simulink model "MPPT_Buck"  (R2022a)
settings: Solver=VariableStepAuto  StartTime=0.0  StopTime=1  RelTol=1e-3
values from neighbouring files (symbols this model uses):
  L = 100e-6    (= 0.0001)    [Boost_Setup.m]
undefined symbols (not defined in the file or in its folder): solarPlant
libraries: spsSeriesRLCBranchLib x4, spsCurrentMeasurementLib x2, slpidlib x2, spsFirstOrderFilterLib x2, spsMosfetLib x2, spsSawtoothGeneratorLib x2, simulink x2, spsMultimeterLib x1, spsPVArrayLib x1, spsVoltageMeasurementLib x1, spspowerguiLib x1
settings Model: Creator=pclem  LastModifiedBy=fion
settings SolverCC: AlgebraicLoopSolver=TrustRegion
settings DebuggingCC: SFMachineParentedDataDiag=warning
settings RTWCC: DLArmComputeVersion=19.05

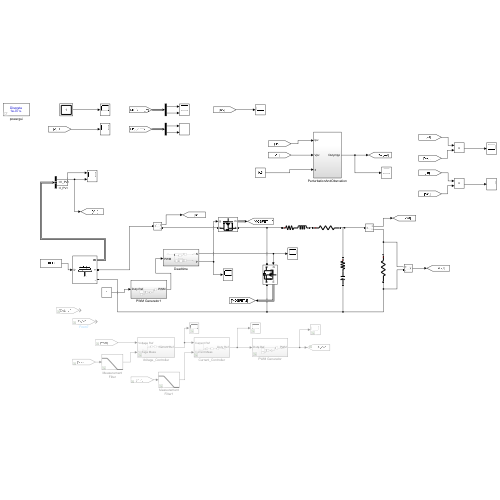
[thumbnail: Simulink's stored preview of the top-level diagram]
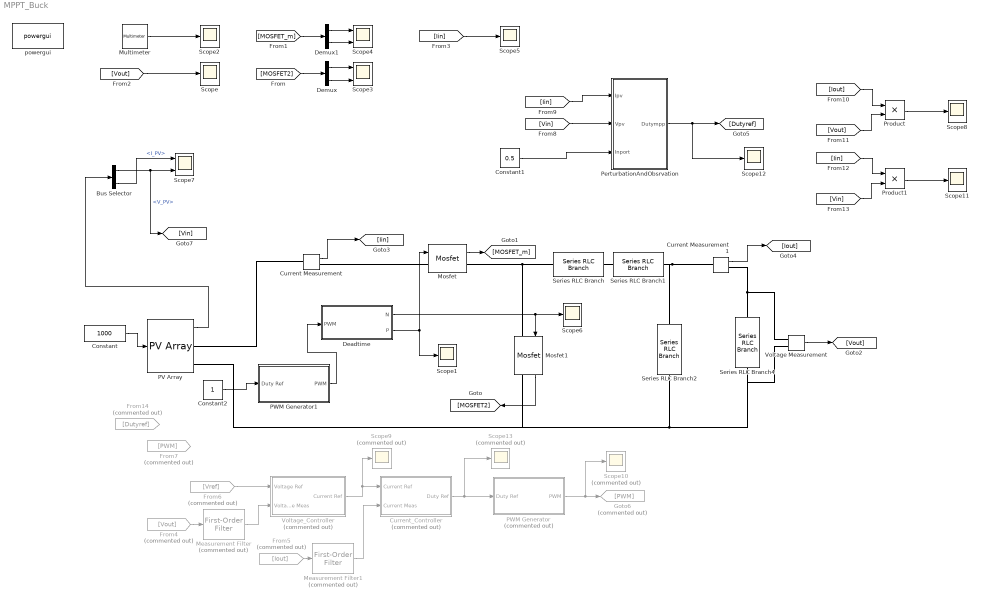
== system MPPT_Buck ==
  Bus Selector : BusSelector  OutputSignals=V_PV,I_PV
  Constant : Constant  Value=1000
  Constant1 : Constant  Value=0.5
  Constant2 : Constant
  Current Measurement : spsCurrentMeasurementLib/Current Measurement  PhasorSimulation=off  OutputType=Complex  PSBequivalent=0
  Current Measurement1 : spsCurrentMeasurementLib/Current Measurement  PhasorSimulation=off  OutputType=Complex  PSBequivalent=0
  Current_Controller : Subsystem  Commented=on
  Deadtime : Subsystem
  Demux : Demux  Outputs=2
  Demux1 : Demux  Outputs=2
  From14 : From  Commented=on  GotoTag=Dutyref
  From4 : From  Commented=on  GotoTag=Vout
  From5 : From  Commented=on  GotoTag=Iout
  From6 : From  Commented=on  GotoTag=Vref
  From7 : From  Commented=on  GotoTag=PWM
  Goto6 : Goto  Commented=on  GotoTag=PWM
  Measurement Filter : spsFirstOrderFilterLib/First-Order Filter  Commented=on  FilterType=Lowpass  Tc=10000*2.2e-9  Ts=0  Initialize=on  Vac_Init=[0, 0, 0]  Vdc_Init=0  PlotResponse=off  FreqRange="[0,  100e3,  100]"
  Measurement Filter1 : spsFirstOrderFilterLib/First-Order Filter  Commented=on  FilterType=Lowpass  Tc=10000*2.2e-9  Ts=0  Initialize=on  Vac_Init=[0, 0, 0]  Vdc_Init=0  PlotResponse=off  FreqRange="[0,  100e3,  100]"
  Mosfet : spsMosfetLib/Mosfet  Ron=0.136  Lon=0  Rd=0.01  Vfd=1.1  IC=0  Rs=1e9  Cs=inf  Measurements=on
  Mosfet1 : spsMosfetLib/Mosfet  Ron=0.136  Lon=0  Rd=0.01  Vfd=1.1  IC=0  Rs=1e9  Cs=inf  Measurements=on
  Multimeter : spsMultimeterLib/Multimeter  L=5  sel=3  yselected={}  Gain=1  OutputType=Complex  PlotAtSimulationStop=off  PhasorSimulation=off
  PV Array : spsPVArrayLib/PV Array  Npar=2  Nser=2  PlotType=array @ 1000 W/m2 & specified temperatures  S_vec="[ 1000  500  100 ]"  Temp_C_vec="[ 45 25  ]"  ModuleName=User-defined  PlotWhenSelected=off  Pm=1.0215  Ncell=2  Voc=5.7  Isc=0.24  Vm=4.5  Im=0.227  beta_Voc_pc=-0.45  alpha_Isc_pc=0.1  beta_Voc=-0.02565  alpha_Isc=0.00024  IL=0.24235  I0=1.5749e-15  nI=3  Rsh=692.3081  Rs=0.0049096  RobustModel=on  RobustCellTemperature=25  BAL=on  Tc=1e-6  Tfilter=5e-5
  PWM Generator : Subsystem  Commented=on
  PWM Generator1 : Subsystem
  PerturbationAndObsrvation : Subsystem  VariantControl=perturbationAndObservation
  Product : Product
  Product1 : Product
  Scope{,1..2,5..6,8,11..12} (8 alike) : Scope
  Scope10 : Scope  Commented=on
  Scope13 : Scope  Commented=on
  Scope3 : Scope  NumInputPorts=2
  Scope4 : Scope  NumInputPorts=2
  Scope7 : Scope  NumInputPorts=2
  Scope9 : Scope  Commented=on
  Series RLC Branch : spsSeriesRLCBranchLib/Series RLC Branch  LConnTagsString=__new0  RConnTagsString=__new0  BranchType=RL  Resistance=25e-3  Inductance=100e-6  SetiL0=off  InitialCurrent=0  Capacitance=1e-6  Setx0=off  InitialVoltage=0  Measurements=Branch current
  Series RLC Branch1 : spsSeriesRLCBranchLib/Series RLC Branch  LConnTagsString=__new0  RConnTagsString=__new0  BranchType=R  Resistance=0.1  Inductance=L  SetiL0=off  InitialCurrent=0  Capacitance=1e-6  Setx0=off  InitialVoltage=0  Measurements=Branch current
  Series RLC Branch2 : spsSeriesRLCBranchLib/Series RLC Branch  LConnTagsString=__new0  RConnTagsString=__new0  BranchType=RC  Resistance=0.1114  Inductance=1e-3  SetiL0=off  InitialCurrent=0  Capacitance=1000e-6  Setx0=off  InitialVoltage=0  Measurements=Branch voltage
  Series RLC Branch4 : spsSeriesRLCBranchLib/Series RLC Branch  LConnTagsString=__new0  RConnTagsString=__new0  BranchType=R  Resistance=10  Inductance=1e-3  SetiL0=off  InitialCurrent=0  Capacitance=1e-6  Setx0=off  InitialVoltage=0  Measurements=Branch voltage and current
  Voltage Measurement : spsVoltageMeasurementLib/Voltage Measurement  PhasorSimulation=off  OutputType=Complex  PSBequivalent=0
  Voltage_Controller : Subsystem  Commented=on
  powergui : spspowerguiLib/powergui  Priority=1  SimulationMode=Discrete  SampleTime=1e-7  frequency=60  Iterations=50  frequencyindice=0  Pbase=100e6  ErrMax=1e-4  UnitsV=kV  UnitsW=MW  buscounter=0  FunctionMessages=off  echomessages=off  EnableUseOfTLC=off  CurrentSourceSwitches=off  DisableSnubberDevices=off  DisableRonSwitches=off  DisableVfSwitches=off  DisplayEquations=off  AutomaticDiscreteSolvers=off  SolverType=Tustin/Backward Euler (TBE)  Interpol=off  ExternalGateDelay=off  methode=off  Ts=100  x0status=blocks  SPID=on  SwTol=0  HookPort=off  NonlinearTolerance=1e-4  nMaxIteration=100  ContinueOnMaxIteration=off  RestoreLinks=warning  ResistiveCurrentMeasurement=off  Frange=[0:2:500]  Ylog=off  Xlog=on  ShowGrid=off  save=off  variable=ZData  structure=0  ZoomFFT=off  StartTime=0.0  cycles=1  DisplayStyle=1  fundamental=60  FreqAxis=off  MaxFrequency=1000  frequencyindicesteady=1  RmsSteady=1  display=off
  wires:
  Multimeter/1 -> Scope2/1
  [Vout] -> Scope/1
  Mosfet/1 -> [MOSFET_m]
  Demux/2 -> Scope3/2
  Demux/1 -> Scope3/1
  [MOSFET2] -> Demux/1
  [MOSFET_m] -> Demux1/1
  Demux1/1 -> Scope4/1
  Demux1/2 -> Scope4/2
  Voltage Measurement/1 -> [Vout]
  Mosfet1/1 -> [MOSFET2]
  Current Measurement/1 -> [Iin]
  [Iin] -> Scope5/1
  Deadtime/2(P) -> Scope1/1, Mosfet/1
  Deadtime/1(N) -> Mosfet1/1, Scope6/1
  Bus Selector/2 -> Scope7/1  "<I_PV>"
  PV Array/1 -> Bus Selector/1
  Bus Selector/1 -> [Vin], Scope7/2  "<V_PV>"
  Constant/1 -> PV Array/1
  Current Measurement1/1 -> [Iout]
  Current_Controller/1(Duty Ref) -> Scope13/1, PWM Generator/1(Duty Ref)
  From5/1 -> Measurement Filter1/1
  Measurement Filter/1 -> Voltage_Controller/2(Voltage Meas)
  Voltage_Controller/1(Current Ref) -> Scope9/1, Current_Controller/1(Current Ref)
  Measurement Filter1/1 -> Current_Controller/2(Current Meas)
  PWM Generator/1(PWM) -> Scope10/1, Goto6/1
  From4/1 -> Measurement Filter/1
  From6/1 -> Voltage_Controller/1(Voltage Ref)
  [Vin] -> PerturbationAndObsrvation/2(Vpv)
  [Iout] -> Product/1
  [Vout] -> Product/2
  Product/1 -> Scope8/1
  Product1/1 -> Scope11/1
  [Vin] -> Product1/2
  [Iin] -> Product1/1
  [Iin] -> PerturbationAndObsrvation/1(Ipv)
  PerturbationAndObsrvation/1(Dutympp) -> Scope12/1, [Dutyref]
  PWM Generator1/1(PWM) -> Deadtime/1(PWM)
  Constant1/1 -> PerturbationAndObsrvation/3(Inport)
  Constant2/1 -> PWM Generator1/1(Duty Ref)
  connections:
  Voltage Measurement/LConn2 -- Series RLC Branch4/RConn1 -- PV Array/RConn2 -- Mosfet1/RConn1 -- Series RLC Branch2/RConn1
  Series RLC Branch1/LConn1 -- Series RLC Branch/RConn1
  Series RLC Branch/LConn1 -- Mosfet/RConn1 -- Mosfet1/LConn1
  Current Measurement/RConn1 -- Mosfet/LConn1
  Current Measurement1/LConn1 -- Series RLC Branch1/RConn1 -- Series RLC Branch2/LConn1
  Voltage Measurement/LConn1 -- Current Measurement1/RConn1 -- Series RLC Branch4/LConn1
  PV Array/RConn1 -- Current Measurement/LConn1

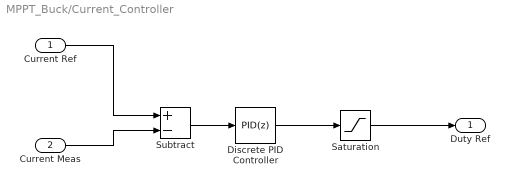
== system MPPT_Buck/Current_Controller ==
  Current Ref : Inport
  Current Meas : Inport  Port=2
  Discrete PID Controller : slpidlib/PID Controller  Controller=PID  Form=Parallel  TimeDomain=Discrete-time  UseExternalTs=off  SampleTime=1/1000  IntegratorMethod=Forward Euler  FilterMethod=Forward Euler  ControllerParametersSource=internal  P=0.02512  I=39.4  UseKiTs=off  D=0  N=100  UseFilter=off  TunerSelectOption=Transfer Function Based (PID Tuner App)  InitialConditionSource=internal  InitialConditionForIntegrator=0  InitialConditionForFilter=0  DifferentiatorICPrevScaledInput=0  ExternalReset=none  TrackingMode=off  Kt=1  LimitOutput=off  SatLimitsSource=internal  UpperSaturationLimit=inf  LowerSaturationLimit=-inf  LinearizeAsGain=off  AntiWindupMode=none  Kb=1  POutMin=[]  POutMax=[]  IOutMin=[]  IOutMax=[]  DOutMin=[]  DOutMax=[]  NOutMin=[]  NOutMax=[]  SumOutMin=[]  SumOutMax=[]  SaturationOutMin=[]  SaturationOutMax=[]  PParamMin=[]  PParamMax=[]  IParamMin=[]  IParamMax=[]  DParamMin=[]  DParamMax=[]  NParamMin=[]  NParamMax=[]  KbParamMin=[]  KbParamMax=[]  KtParamMin=[]  KtParamMax=[]  KbOutMin=[]  KbOutMax=[]  KtOutMin=[]  KtOutMax=[]  IntegratorOutMin=[]  IntegratorOutMax=[]  FilterOutMin=[]  FilterOutMax=[]  SumI1OutMin=[]  SumI1OutMax=[]  SumI2OutMin=[]  SumI2OutMax=[]  SumI3OutMin=[]  SumI3OutMax=[]  SumI4OutMin=[]  SumI4OutMax=[]  SumDOutMin=[]  SumDOutMax=[]  DifferentiatorOutMin=[]  DifferentiatorOutMax=[]  FilterDiffOutCoefMin=[]  FilterDiffOutCoefMax=[]  ReciprocalOutMin=[]  ReciprocalOutMax=[]  SumDenOutMin=[]  SumDenOutMax=[]  SumNumOutMin=[]  SumNumOutMax=[]  DivideOutMin=[]  DivideOutMax=[]  UdiffTsProdOutMin=[]  UdiffTsProdOutMax=[]  NTsProdOutMin=[]  NTsProdOutMax=[]  UintegralTsProdOutMin=[]  UintegralTsProdOutMax=[]  UngainTsProdOutMin=[]  UngainTsProdOutMax=[]  IntegratorContinuousStateAttributes=''  IntegratorStateMustResolveToSignalObject=off  IntegratorRTWStateStorageClass=Auto  FilterContinuousStateAttributes=''  FilterStateMustResolveToSignalObject=off  FilterRTWStateStorageClass=Auto  ParallelPVariant=InternalParameters  IdealPVariant=Disabled  IVariant=InternalParameters  DVariant=InternalParameters  IntegratorVariant=Discrete  SatVariant=Disabled  AWVariant=Passthrough  PCopyVariant=Disabled  TRVariant=Disabled  FdbkBlocksVariant=Forward  IdealPFdbkVariant=Disabled  SatFdbkVariant=Disabled  DerivativeFilterVariant=Differentiator  NVariant=Passthrough  NCopyVariant=Disabled_SignalSpec  FilterICVariant=InternalICsDifferentiator  IntegratorICVariant=InternalICs  ExternalResetVariant=Disabled  TRSumVariant=Passthrough  SumFdbkVariant=Disabled  SumVariant=Sum_PID  TsampFilterVariant=InternalTs  TsampNgainVariant=Passthrough  TsampIntegralVariant=Passthrough  ExternalSaturationOutDataTypeStr=Inherit: Same as second input  aMode=0
  Saturation : Saturate  UpperLimit=0.98  LowerLimit=0.02
  Subtract : Sum  Inputs=+-
  Duty Ref : Outport
  wires:
  Subtract/1 -> Discrete PID Controller/1
  Saturation/1 -> Duty Ref/1
  Current Meas/1 -> Subtract/2
  Discrete PID Controller/1 -> Saturation/1
  Current Ref/1 -> Subtract/1

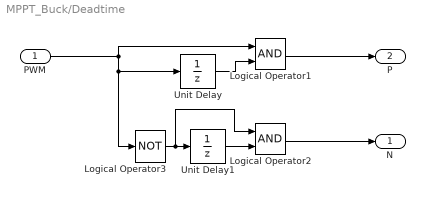
== system MPPT_Buck/Deadtime ==
  PWM : Inport
  Logical Operator1 : Logic  AllPortsSameDT=off  OutDataTypeStr=boolean
  Logical Operator2 : Logic  AllPortsSameDT=off  OutDataTypeStr=boolean
  Logical Operator3 : Logic  Operator=NOT  AllPortsSameDT=off  OutDataTypeStr=boolean
  Unit Delay : UnitDelay  SampleTime=-1  HasFrameUpgradeWarning=on
  Unit Delay1 : UnitDelay  SampleTime=-1  HasFrameUpgradeWarning=on
  N : Outport
  P : Outport  Port=2
  wires:
  Logical Operator1/1 -> P/1
  Logical Operator2/1 -> N/1
  Unit Delay1/1 -> Logical Operator2/2
  PWM/1 -> Logical Operator1/1, Unit Delay/1, Logical Operator3/1
  Logical Operator3/1 -> Unit Delay1/1, Logical Operator2/1
  Unit Delay/1 -> Logical Operator1/2

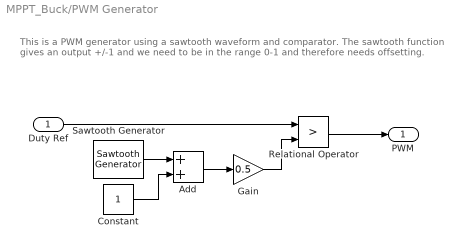
== system MPPT_Buck/PWM Generator ==
  note: This is a PWM generator using a sawtooth waveform and comparator.
      |
      | The sawtooth function gives an output +/-1 and we need to be in the range 0-1 and therefore needs offsetting.
  Duty Ref : Inport
  Add : Sum
  Constant : Constant
  Gain : Gain  Gain=0.5
  Relational Operator : RelationalOperator  Operator=>  OutDataTypeStr=boolean  RndMeth=Simplest  InputSameDT=off
  Sawtooth Generator : spsSawtoothGeneratorLib/Sawtooth Generator  Freq=62500  Phase=180  Ts=1e-7
  PWM : Outport
  wires:
  Duty Ref/1 -> Relational Operator/1
  Relational Operator/1 -> PWM/1
  Constant/1 -> Add/2
  Add/1 -> Gain/1
  Sawtooth Generator/1 -> Add/1
  Gain/1 -> Relational Operator/2

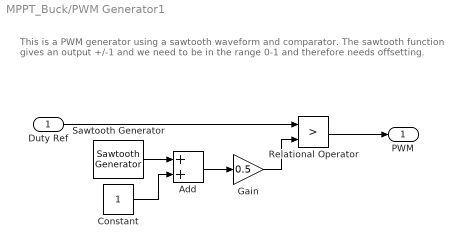
== system MPPT_Buck/PWM Generator1 ==
  note: This is a PWM generator using a sawtooth waveform and comparator.
      |
      | The sawtooth function gives an output +/-1 and we need to be in the range 0-1 and therefore needs offsetting.
  Duty Ref : Inport
  Add : Sum
  Constant : Constant
  Gain : Gain  Gain=0.5
  Relational Operator : RelationalOperator  Operator=>  OutDataTypeStr=boolean  RndMeth=Simplest  InputSameDT=off
  Sawtooth Generator : spsSawtoothGeneratorLib/Sawtooth Generator  Freq=62500  Phase=180  Ts=1e-7
  PWM : Outport
  wires:
  Gain/1 -> Relational Operator/2
  Sawtooth Generator/1 -> Add/1
  Add/1 -> Gain/1
  Constant/1 -> Add/2
  Relational Operator/1 -> PWM/1
  Duty Ref/1 -> Relational Operator/1

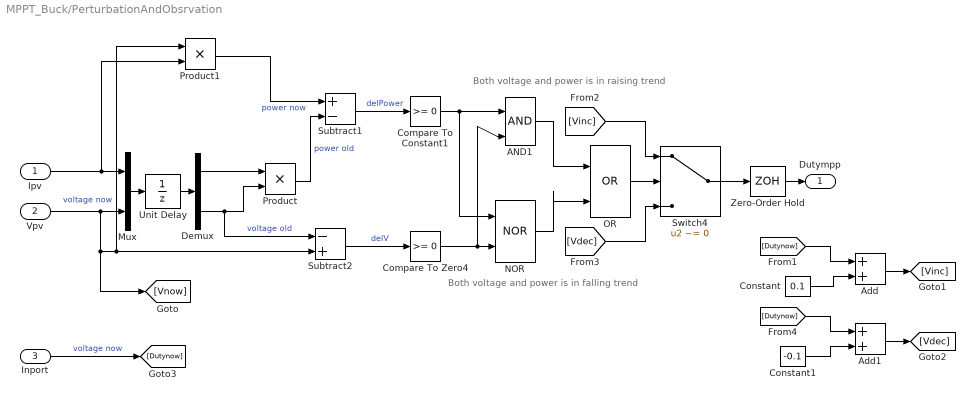
== system MPPT_Buck/PerturbationAndObsrvation ==
  note: Both voltage and power is in falling trend
  note: Both voltage and power is in raising trend
  Ipv : Inport
  Vpv : Inport  Port=2
  Inport : Inport  Port=3
  AND1 : Logic  IconShape=distinctive  AllPortsSameDT=off  OutDataTypeStr=boolean
  Add : Sum
  Add1 : Sum
  Compare To Constant1 : simulink/Logic and Bit Operations/Compare To Constant  relop=>=  const=0  OutDataTypeStr=boolean
  Compare To Zero4 : simulink/Logic and Bit Operations/Compare To Zero  relop=>=  OutDataTypeStr=boolean
  Constant : Constant  Value=0.1
  Constant1 : Constant  Value=-0.1
  Demux : Demux  Outputs=2
  Mux : Mux  Inputs=2
  NOR : Logic  Operator=NOR  IconShape=distinctive  AllPortsSameDT=off  OutDataTypeStr=boolean
  OR : Logic  Operator=OR  IconShape=distinctive  AllPortsSameDT=off  OutDataTypeStr=boolean
  Product : Product
  Product1 : Product
  Subtract1 : Sum  Inputs=+-
  Subtract2 : Sum  Inputs=-+
  Switch4 : Switch  Criteria=u2 ~= 0  SaturateOnIntegerOverflow=off  InputSameDT=off
  Unit Delay : UnitDelay  InitialCondition=solarPlant.startMPPTValue  SampleTime=solarPlant.timeMPPT  HasFrameUpgradeWarning=on
  Zero-Order Hold : ZeroOrderHold  SampleTime=20e-3
  Dutympp : Outport  VectorParamsAs1DForOutWhenUnconnected=off
  wires:
  Mux/1 -> Unit Delay/1
  Ipv/1 -> Product1/2, Mux/1
  Demux/1 -> Product/1
  Unit Delay/1 -> Demux/1
  Demux/2 -> Subtract2/1, Product/2  "voltage old"
  Vpv/1 -> [Vnow], Product1/1, Subtract2/2, Mux/2  "voltage now"
  Zero-Order Hold/1 -> Dutympp/1
  [Vinc] -> Switch4/1
  Compare To Constant1/1 -> AND1/1, NOR/1
  [Vdec] -> Switch4/3
  NOR/1 -> OR/2
  Subtract2/1 -> Compare To Zero4/1  "delV"
  Compare To Zero4/1 -> AND1/2, NOR/2
  OR/1 -> Switch4/2
  AND1/1 -> OR/1
  Subtract1/1 -> Compare To Constant1/1  "delPower"
  Switch4/1 -> Zero-Order Hold/1
  Product/1 -> Subtract1/2  "power old"
  Product1/1 -> Subtract1/1  "power now"
  [Dutynow] -> Add/1
  Constant/1 -> Add/2
  Add/1 -> [Vinc]
  Add1/1 -> [Vdec]
  Constant1/1 -> Add1/2
  [Dutynow] -> Add1/1
  Inport/1 -> [Dutynow]  "voltage now"

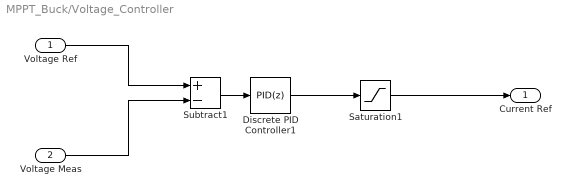
== system MPPT_Buck/Voltage_Controller ==
  Voltage Ref : Inport
  Voltage Meas : Inport  Port=2
  Discrete PID Controller1 : slpidlib/PID Controller  Controller=PID  Form=Parallel  TimeDomain=Discrete-time  UseExternalTs=off  SampleTime=1/1000  IntegratorMethod=Forward Euler  FilterMethod=Forward Euler  ControllerParametersSource=internal  P=0.05024  I=15.78  UseKiTs=off  D=0  N=100  UseFilter=off  TunerSelectOption=Transfer Function Based (PID Tuner App)  InitialConditionSource=internal  InitialConditionForIntegrator=0  InitialConditionForFilter=0  DifferentiatorICPrevScaledInput=0  ExternalReset=none  TrackingMode=off  Kt=1  LimitOutput=off  SatLimitsSource=internal  UpperSaturationLimit=inf  LowerSaturationLimit=-inf  LinearizeAsGain=off  AntiWindupMode=none  Kb=1  POutMin=[]  POutMax=[]  IOutMin=[]  IOutMax=[]  DOutMin=[]  DOutMax=[]  NOutMin=[]  NOutMax=[]  SumOutMin=[]  SumOutMax=[]  SaturationOutMin=[]  SaturationOutMax=[]  PParamMin=[]  PParamMax=[]  IParamMin=[]  IParamMax=[]  DParamMin=[]  DParamMax=[]  NParamMin=[]  NParamMax=[]  KbParamMin=[]  KbParamMax=[]  KtParamMin=[]  KtParamMax=[]  KbOutMin=[]  KbOutMax=[]  KtOutMin=[]  KtOutMax=[]  IntegratorOutMin=[]  IntegratorOutMax=[]  FilterOutMin=[]  FilterOutMax=[]  SumI1OutMin=[]  SumI1OutMax=[]  SumI2OutMin=[]  SumI2OutMax=[]  SumI3OutMin=[]  SumI3OutMax=[]  SumI4OutMin=[]  SumI4OutMax=[]  SumDOutMin=[]  SumDOutMax=[]  DifferentiatorOutMin=[]  DifferentiatorOutMax=[]  FilterDiffOutCoefMin=[]  FilterDiffOutCoefMax=[]  ReciprocalOutMin=[]  ReciprocalOutMax=[]  SumDenOutMin=[]  SumDenOutMax=[]  SumNumOutMin=[]  SumNumOutMax=[]  DivideOutMin=[]  DivideOutMax=[]  UdiffTsProdOutMin=[]  UdiffTsProdOutMax=[]  NTsProdOutMin=[]  NTsProdOutMax=[]  UintegralTsProdOutMin=[]  UintegralTsProdOutMax=[]  UngainTsProdOutMin=[]  UngainTsProdOutMax=[]  IntegratorContinuousStateAttributes=''  IntegratorStateMustResolveToSignalObject=off  IntegratorRTWStateStorageClass=Auto  FilterContinuousStateAttributes=''  FilterStateMustResolveToSignalObject=off  FilterRTWStateStorageClass=Auto  ParallelPVariant=InternalParameters  IdealPVariant=Disabled  IVariant=InternalParameters  DVariant=InternalParameters  IntegratorVariant=Discrete  SatVariant=Disabled  AWVariant=Passthrough  PCopyVariant=Disabled  TRVariant=Disabled  FdbkBlocksVariant=Forward  IdealPFdbkVariant=Disabled  SatFdbkVariant=Disabled  DerivativeFilterVariant=Differentiator  NVariant=Passthrough  NCopyVariant=Disabled_SignalSpec  FilterICVariant=InternalICsDifferentiator  IntegratorICVariant=InternalICs  ExternalResetVariant=Disabled  TRSumVariant=Passthrough  SumFdbkVariant=Disabled  SumVariant=Sum_PID  TsampFilterVariant=InternalTs  TsampNgainVariant=Passthrough  TsampIntegralVariant=Passthrough  ExternalSaturationOutDataTypeStr=Inherit: Same as second input  aMode=0
  Saturation1 : Saturate  UpperLimit=2  LowerLimit=0
  Subtract1 : Sum  Inputs=+-
  Current Ref : Outport
  wires:
  Saturation1/1 -> Current Ref/1
  Subtract1/1 -> Discrete PID Controller1/1
  Voltage Ref/1 -> Subtract1/1
  Discrete PID Controller1/1 -> Saturation1/1
  Voltage Meas/1 -> Subtract1/2
